simulink model "SuspentionModel"  (R2018b)
settings: Solver=VariableStepAuto  StartTime=0.0  StopTime=10.0  RelTol=1e-3
values from neighbouring files (symbols this model uses):
  csc = 600    [SetCoefficients.m]    (also in SetCoefficients_QC.m)
  cse = 1200    [SetCoefficients.m]    (also in SetCoefficients_QC.m)
  ks = 2e4    (= 20000)    [SetCoefficients.m]    (also in SetCoefficients_QC.m)
  ksstiff = 20*ks    (= 400000)    [SetCoefficients.m]    (also in SetCoefficients_QC.m)
  s1 = 0    [Part1_Graphs.m]
  s1d = 1    [Part1_Graphs.m]
  s2 = 0    [Part1_Graphs.m]
  s2d = 0    [Part1_Graphs.m]
  x1 = 0.2    [SetCoefficients.m]    (also in SetCoefficients_QC.m)
  x2 = 0.5    [SetCoefficients.m]    (also in SetCoefficients_QC.m)
settings Model: Creator=joebe  LastModifiedBy=joebe

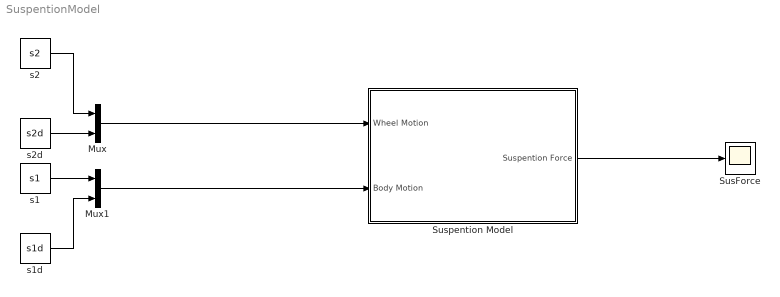
== system SuspentionModel ==
  Mux : Mux  Inputs=2
  Mux1 : Mux  Inputs=2
  SusForce : Scope
  Suspention Model : Subsystem
  s1 : Constant  Value=s1
  s1d : Constant  Value=s1d
  s2 : Constant  Value=s2
  s2d : Constant  Value=s2d
  wires:
  Mux/1 -> Suspention Model/1(Wheel Motion)
  Mux1/1 -> Suspention Model/2(Body Motion)
  s1d/1 -> Mux1/2
  s1/1 -> Mux1/1
  s2d/1 -> Mux/2
  s2/1 -> Mux/1
  Suspention Model/1(Suspention Force) -> SusForce/1

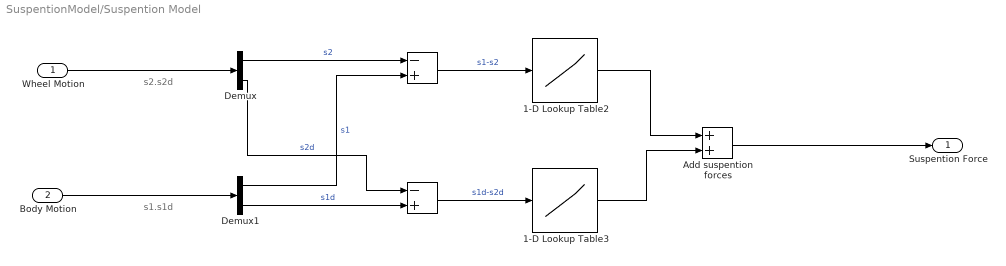
== system SuspentionModel/Suspention Model ==
  note: s1.s1d
  note: s2.s2d
  Wheel Motion : Inport
  Body Motion : Inport  Port=2
  " " : Sum  Inputs=-+
  " " : Sum  Inputs=-+
  1-D Lookup Table2 : Lookup_n-D  NumberOfTableDimensions=1  BreakpointsForDimension1=[-x2 -x1 x1 x2]  Table=[-(ksstiff*(x2-x1)+ks*x1) -x1*ks x1*ks (ksstiff*(x2-x1)+ks*x1)]  InternalRulePriority=Speed  RndMeth=Simplest  InputSameDT=on
  1-D Lookup Table3 : Lookup_n-D  NumberOfTableDimensions=1  BreakpointsForDimension1=[-10 0 10]  Table=[-10*cse 0 10*csc]  InternalRulePriority=Speed  RndMeth=Simplest  InputSameDT=on
  Add suspention forces : Sum
  Demux : Demux  Outputs=2
  Demux1 : Demux  Outputs=2
  Suspention Force : Outport
  wires:
  Demux1/2 -> " "/2  "s1d"
  " "/1 -> 1-D Lookup Table2/1  "s1-s2"
  Demux1/1 -> " "/2  "s1"
  1-D Lookup Table3/1 -> Add suspention forces/2
  1-D Lookup Table2/1 -> Add suspention forces/1
  Demux/1 -> " "/1  "s2"
  Demux/2 -> " "/1  "s2d"
  Body Motion/1 -> Demux1/1
  " "/1 -> 1-D Lookup Table3/1  "s1d-s2d"
  Add suspention forces/1 -> Suspention Force/1
  Wheel Motion/1 -> Demux/1
